simulink model "gnss_receiver"  (R2020b)
settings: Solver=VariableStepAuto  StartTime=0.0  StopTime=10.0  RelTol=1e-3
model mask{fix=3, num_sat=16, pos_acc_m=[0 0 0], vel_acc_mps=[0 0 0], sample_rate=5}
  mask prompts: fix "Fix (0 = No Fix, 1 = Time Only, 2 = 2D, 3 = 3D"; num_sat "Number of Satellites:"; pos_acc_m "Position Accuracy [m]:"; vel_acc_mps "Velocity Accuracy [m]:"; sample_rate "Sample Rate [Hz]:"
model workspace (MAT data in the model file):
  fix = Simulink.Parameter
  fix.Value = 3
  fix.DataType = 'auto'
  fix.Dimensions = [1 1]
  num_sat = Simulink.Parameter
  num_sat.Value = 16
  num_sat.DataType = 'auto'
  num_sat.Dimensions = [1 1]
  pos_acc_m = Simulink.Parameter
  pos_acc_m.Value = [0 0 0]
  pos_acc_m.DataType = 'auto'
  pos_acc_m.Dimensions = [1 3]
  sample_rate = Simulink.Parameter
  sample_rate.Value = 5
  sample_rate.DataType = 'auto'
  sample_rate.Dimensions = [1 1]
  vel_acc_mps = Simulink.Parameter
  vel_acc_mps.Value = [0 0 0]
  vel_acc_mps.DataType = 'auto'
  vel_acc_mps.Dimensions = [1 3]
undefined symbols (not defined in the file): datetime, datevec, Earth, WGS84
libraries: simulink x2, aerolibconvert2 x2, aerolibtransform2 x1
settings Model: ParameterArgumentNames=fix,num_sat,pos_acc_m,sample_rate,vel_acc_mps  OrderedModelArguments=off  Creator=brian  LastModifiedBy=brian

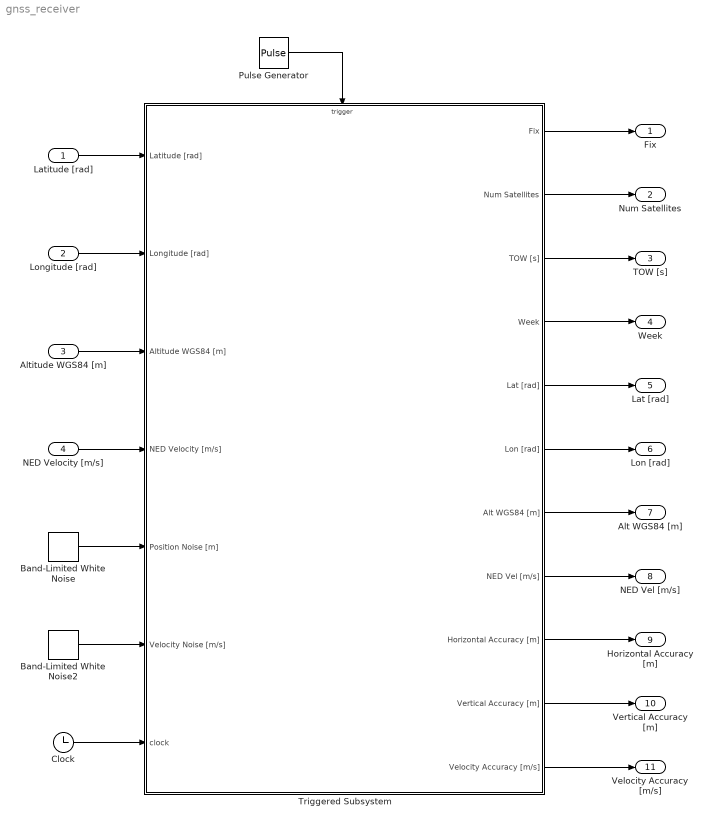
== system gnss_receiver ==
  Latitude [rad] : Inport
  "Longitude [rad] " : Inport  Port=2
  Altitude WGS84 [m] : Inport  Port=3
  NED Velocity [m/s] : Inport  Port=4
  Band-Limited White Noise : simulink/Sources/Band-Limited White Noise  Cov=pos_acc_m  Ts=0.1  seed=[23341]
  Band-Limited White Noise2 : simulink/Sources/Band-Limited White Noise  Cov=vel_acc_mps  Ts=0.1  seed=[23341]
  Clock : Clock
  Pulse Generator : DiscretePulseGenerator  PulseType=Time based  Period=1/sample_rate  PulseWidth=5
  Triggered Subsystem : Subsystem  TreatAsAtomicUnit=on
  Fix : Outport
  Num Satellites : Outport  Port=2
  TOW [s] : Outport  Port=3
  Week : Outport  Port=4
  Lat [rad] : Outport  Port=5
  Lon [rad] : Outport  Port=6
  Alt WGS84 [m] : Outport  Port=7
  NED Vel [m/s] : Outport  Port=8
  Horizontal Accuracy [m] : Outport  Port=9
  Vertical Accuracy [m] : Outport  Port=10
  Velocity Accuracy [m/s] : Outport  Port=11
  wires:
  Triggered Subsystem/10(Vertical Accuracy [m]) -> Vertical Accuracy [m]/1
  Pulse Generator/1 -> Triggered Subsystem/Trigger
  Triggered Subsystem/1(Fix) -> Fix/1
  Clock/1 -> Triggered Subsystem/7(clock)
  Triggered Subsystem/11(Velocity Accuracy [m/s]) -> Velocity Accuracy [m/s]/1
  Triggered Subsystem/5(Lat [rad]) -> Lat [rad]/1
  NED Velocity [m/s]/1 -> Triggered Subsystem/4(NED Velocity [m/s])
  Triggered Subsystem/9(Horizontal Accuracy [m]) -> Horizontal Accuracy [m]/1
  Altitude WGS84 [m]/1 -> Triggered Subsystem/3(Altitude WGS84 [m])
  Triggered Subsystem/3(TOW [s]) -> TOW [s]/1
  Latitude [rad]/1 -> Triggered Subsystem/1(Latitude [rad])
  "Longitude [rad] "/1 -> Triggered Subsystem/2("Longitude [rad] ")
  Triggered Subsystem/7(Alt WGS84 [m]) -> Alt WGS84 [m]/1
  Triggered Subsystem/8(NED Vel [m/s]) -> NED Vel [m/s]/1
  Band-Limited White Noise2/1 -> Triggered Subsystem/6(Velocity Noise [m/s])
  Triggered Subsystem/4(Week) -> Week/1
  Triggered Subsystem/2(Num Satellites) -> Num Satellites/1
  Triggered Subsystem/6(Lon [rad]) -> Lon [rad]/1
  Band-Limited White Noise/1 -> Triggered Subsystem/5(Position Noise [m])

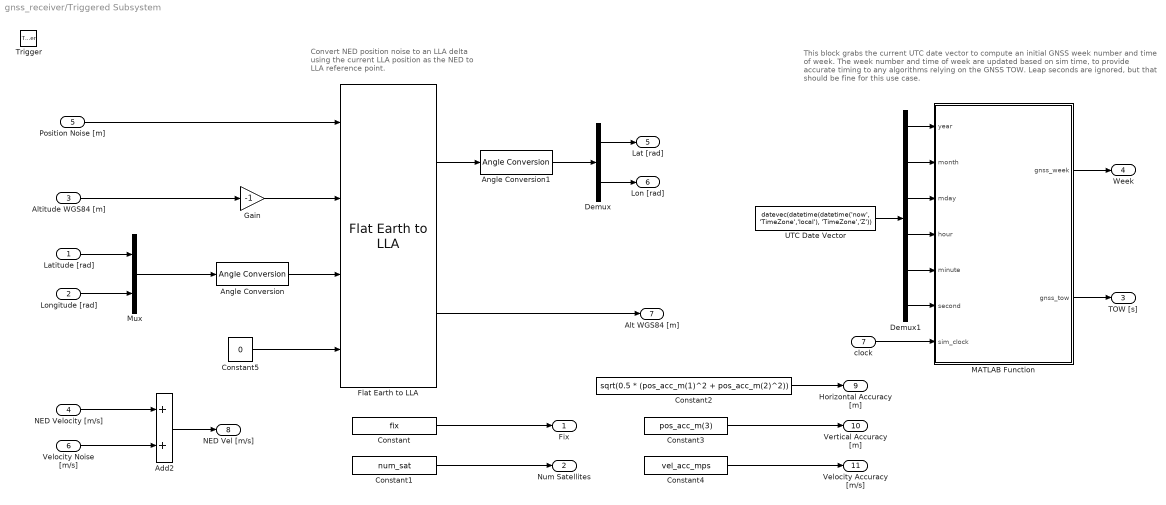
== system gnss_receiver/Triggered Subsystem ==
  note: This block grabs the current UTC date vector to compute an initial GNSS week number
      | and time of week. The week number and time of week are updated based on sim time, to provide accurate timing to any algorithms relying on the GNSS TOW. Leap seconds are ignored, but that should be fine for this use case.
  note: Convert NED position noise to an LLA delta
      | using the current LLA position as the NED to
      | LLA reference point.
  Latitude [rad] : Inport
  "Longitude [rad] " : Inport  Port=2
  Altitude WGS84 [m] : Inport  Port=3
  NED Velocity [m/s] : Inport  Port=4  PortDimensions=3
  Position Noise [m] : Inport  Port=5  PortDimensions=3
  Velocity Noise [m/s] : Inport  Port=6  PortDimensions=3
  clock : Inport  Port=7
  Trigger : TriggerPort  VariantControl=Variant
  Add2 : Sum
  Angle Conversion : aerolibconvert2/Angle Conversion  IU=rad  OU=deg
  Angle Conversion1 : aerolibconvert2/Angle Conversion  IU=deg  OU=rad
  Constant : Constant  Value=fix
  Constant1 : Constant  Value=num_sat
  Constant2 : Constant  Value=sqrt(0.5 * (pos_acc_m(1)^2 + pos_acc_m(2)^2))
  Constant3 : Constant  Value=pos_acc_m(3)
  Constant4 : Constant  Value=vel_acc_mps
  Constant5 : Constant  Value=0
  Demux : Demux  Outputs=2
  Demux1 : Demux  Outputs=6
  Flat Earth to LLA : aerolibtransform2/Flat Earth to LLA  units=Metric (MKS)  ptype=Earth (WGS84)  F=1/298.257223563  R=6378137  refPosPort=on  LL0=[0 10]  psi=0
  Gain : Gain  Gain=-1
  MATLAB Function : MATLAB Function  TreatAsAtomicUnit=on
  Mux : Mux  Inputs=2
  UTC Date Vector : Constant  Value=datevec(datetime(datetime('now', 'TimeZone','local'), 'TimeZone','Z'))  SampleTime=-1
  Fix : Outport
  Num Satellites : Outport  Port=2
  TOW [s] : Outport  Port=3
  Week : Outport  Port=4
  Lat [rad] : Outport  Port=5
  Lon [rad] : Outport  Port=6
  Alt WGS84 [m] : Outport  Port=7
  NED Vel [m/s] : Outport  Port=8
  Horizontal Accuracy [m] : Outport  Port=9
  Vertical Accuracy [m] : Outport  Port=10
  Velocity Accuracy [m/s] : Outport  Port=11
  wires:
  Constant/1 -> Fix/1
  Constant1/1 -> Num Satellites/1
  Constant2/1 -> Horizontal Accuracy [m]/1
  Constant3/1 -> Vertical Accuracy [m]/1
  Constant4/1 -> Velocity Accuracy [m/s]/1
  Position Noise [m]/1 -> Flat Earth to LLA/1
  Altitude WGS84 [m]/1 -> Gain/1
  Mux/1 -> Angle Conversion/1
  Angle Conversion/1 -> Flat Earth to LLA/3
  Constant5/1 -> Flat Earth to LLA/4
  "Longitude [rad] "/1 -> Mux/2
  Latitude [rad]/1 -> Mux/1
  Flat Earth to LLA/1 -> Angle Conversion1/1
  Angle Conversion1/1 -> Demux/1
  Demux/2 -> Lon [rad]/1
  Demux/1 -> Lat [rad]/1
  Flat Earth to LLA/2 -> Alt WGS84 [m]/1
  NED Velocity [m/s]/1 -> Add2/1
  Velocity Noise [m/s]/1 -> Add2/2
  Add2/1 -> NED Vel [m/s]/1
  Demux1/2 -> MATLAB Function/2(month)
  Demux1/6 -> MATLAB Function/6(second)
  UTC Date Vector/1 -> Demux1/1
  Demux1/1 -> MATLAB Function/1(year)
  Demux1/5 -> MATLAB Function/5(minute)
  Demux1/4 -> MATLAB Function/4(hour)
  Demux1/3 -> MATLAB Function/3(mday)
  MATLAB Function/2(gnss_tow) -> TOW [s]/1
  MATLAB Function/1(gnss_week) -> Week/1
  clock/1 -> MATLAB Function/7(sim_clock)
  Gain/1 -> Flat Earth to LLA/2

== matlab function gnss_receiver/Triggered Subsystem/MATLAB Function ==
  data: year input; month input; mday input; hour input; minute input; second input; gnss_week output; sim_clock input; gnss_tow output
function [gnss_week, gnss_tow] = GnssWeekAndTime(year, month, mday, hour, minute, second, sim_clock)

JAN61980 = 44244;
JAN11901 = 15385;
SEC_PER_DAY = 86400.0;

month_day = [
    0, 31, 59, 90, 120, 151, 181, 212, 243, 273, 304, 334;
    0, 31, 60, 91, 121, 152, 182, 213, 244, 274, 305, 335
];

second = second + sim_clock;
leap = (mod(year,4) == 0);
yday = month_day(leap + 1, month) + mday;
mjd = ((year - 1901) / 4) * 1461 + mod((year - 1901), 4) * 365 + yday - 1 + JAN11901;
fmjd = ((second / 60.0 + minute) / 60.0 + hour) / 24.0;
gnss_week = floor((mjd - JAN61980) / 7);
gnss_tow = ((mjd - JAN61980) - gnss_week * 7 + fmjd) * SEC_PER_DAY;
